simulink model "ecusimu"  (R2015a)
settings: Solver=ode45  StartTime=0.0  StopTime=inf  RelTol=1e-3
libraries: dsparch4 x6, dspsrcs4 x1, dspvision x1, dspsnks4 x1
settings Model: Creator=lina  LastModifiedBy=lina

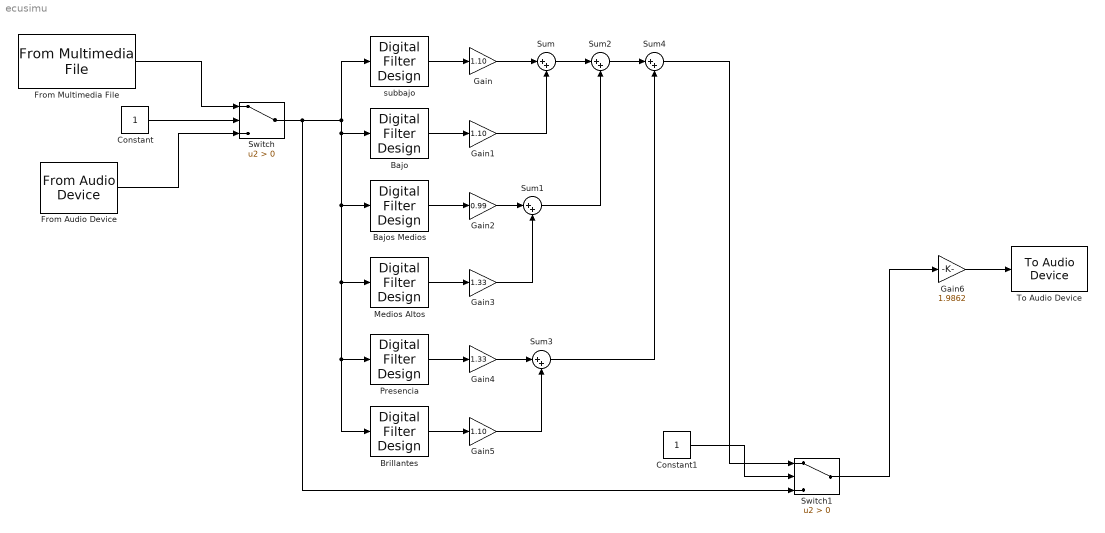
== system ecusimu ==
  Bajo : dsparch4/Digital Filter Design  mwdsp_browser_bugfix_var=off
  Bajos Medios : dsparch4/Digital Filter Design  mwdsp_browser_bugfix_var=off
  Brillantes : dsparch4/Digital Filter Design  mwdsp_browser_bugfix_var=off
  Constant : Constant  VectorParams1D=off
  Constant1 : Constant
  From Audio Device : dspsrcs4/From Audio Device  deviceName=Default  numChannels=2  sampleRate=44100  deviceDatatype=16-bit integer  autoBufferSize=on  bufferSize=4096  queueDuration=1.0  frameSize=1024  outputDatatype=double  defaultInputChannelMapping=on  inputChannelMapping=1:2  outputNumOverrunSamples=off
  From Multimedia File : dspvision/From Multimedia File  inputFilename=E:\universidad\DSP 1\ecualizador\Serj Tankian - Harakiri.wav  loop=on  numPlays=inf  outputStreams=Audio only  videoDataType=single  audioDataType=double  inheritSampleTime=on  userDefinedSampleTime=1/30  noAudioOutput=off  isIntensityVideo=off  fourcc=RGB  colorVideoFormat=Separate color signals  outputEOF=off  dataOrg=Column-major  audioFrameSize=1024  computeAudioFrameSize=off  outSamplingMode=Sample based
  Gain : Gain  Gain=1.10
  Gain1 : Gain  Gain=1.10
  Gain2 : Gain  Gain=0.99
  Gain3 : Gain  Gain=1.33
  Gain4 : Gain  Gain=1.33
  Gain5 : Gain  Gain=1.10
  Gain6 : Gain  Gain=1.9862
  Medios Altos : dsparch4/Digital Filter Design  mwdsp_browser_bugfix_var=off
  Presencia : dsparch4/Digital Filter Design  mwdsp_browser_bugfix_var=off
  Sum{,1..4} (5 alike) : Sum  Inputs=|++
  Switch : Switch  Criteria=u2 > Threshold
  Switch1 : Switch  Criteria=u2 > Threshold
  To Audio Device : dspsnks4/To Audio Device  deviceName=Default  inheritSampleRate=on  sampleRate=44100  deviceDatatype=Determine from input data type  autoBufferSize=on  bufferSize=4096  queueDuration=1.0  defaultOutputChannelMapping=on  outputChannelMapping=1:2  outputNumUnderrunSamples=off
  subbajo : dsparch4/Digital Filter Design  mwdsp_browser_bugfix_var=off
  wires:
  From Audio Device/1 -> Switch/3
  From Multimedia File/1 -> Switch/1
  Constant/1 -> Switch/2
  Switch/1 -> Switch1/3, Presencia/1, Brillantes/1, Medios Altos/1, Bajos Medios/1, Bajo/1, subbajo/1
  subbajo/1 -> Gain/1
  Bajo/1 -> Gain1/1
  Gain/1 -> Sum/1
  Gain1/1 -> Sum/2
  Bajos Medios/1 -> Gain2/1
  Medios Altos/1 -> Gain3/1
  Gain2/1 -> Sum1/1
  Gain3/1 -> Sum1/2
  Sum/1 -> Sum2/1
  Sum1/1 -> Sum2/2
  Brillantes/1 -> Gain5/1
  Presencia/1 -> Gain4/1
  Gain4/1 -> Sum3/1
  Gain5/1 -> Sum3/2
  Sum2/1 -> Sum4/1
  Sum3/1 -> Sum4/2
  Gain6/1 -> To Audio Device/1
  Sum4/1 -> Switch1/1
  Constant1/1 -> Switch1/2
  Switch1/1 -> Gain6/1
